simulink model "P3"  (R2017b)
settings: Solver=VariableStepAuto  StartTime=0.0  StopTime=10.0  RelTol=1e-3
undefined symbols (not defined in the file): b, g, I, l, m_p, m_t
settings Model: Creator=Stephen  LastModifiedBy=Stephen

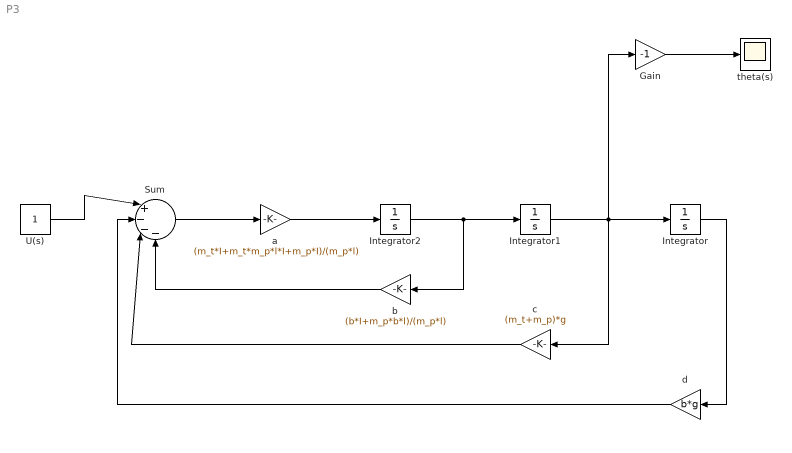
== system P3 ==
  Gain : Gain  Gain=-1
  Integrator : Integrator
  Integrator1 : Integrator
  Integrator2 : Integrator
  Sum : Sum  Inputs=|+---
  U(s) : Constant
  a : Gain  Gain=(m_t*I+m_t*m_p*l*I+m_p*I)/(m_p*l)
  b : Gain  Gain=(b*I+m_p*b*l)/(m_p*l)
  c : Gain  Gain=(m_t+m_p)*g
  d : Gain  Gain=b*g
  theta(s) : Scope
  wires:
  Sum/1 -> a/1
  a/1 -> Integrator2/1
  Integrator2/1 -> b/1, Integrator1/1
  Integrator1/1 -> Gain/1, c/1, Integrator/1
  Integrator/1 -> d/1
  b/1 -> Sum/4
  c/1 -> Sum/3
  d/1 -> Sum/2
  Gain/1 -> theta(s)/1
  U(s)/1 -> Sum/1
